simulink model "mdl_example_7_2"  (R2024b)
settings: Solver=FixedStepAuto  StartTime=0.0  StopTime=20*60  FixedStep=1e-2  RelTol=1e-3
values from neighbouring files (symbols this model uses):
  Cd = diag([kd kd kd])    [example_7_2_init.m]
  hw0_B = [0 0 0]'    [example_7_2_init.m]
  inv_qc = inv_q(qc)    [example_7_2_init.m]
  J2 = [6400  -76.4    -25.6 ... (first row only)    [example_7_2_init.m]
  kp = 10    [example_7_2_init.m]
  q0 = (sqrt(2)/2)*[1 0 0 1]'    [example_7_2_init.m]
  w0 = [0.01 0.01 0.01]'    [example_7_2_init.m]
  W4 = (1/sqrt(2))*W4    [example_7_2_init.m]
  W4_inv = pinv(W4)    [example_7_2_init.m]
  WN = [1 0 0 1/sqrt(3) ... (first row only)    [example_7_2_init.m]
  WN_inv = pinv(WN)    [example_7_2_init.m]
libraries: aerolibutil x1
settings Model: SimulationMode=accelerator  Creator=Monster  LastModifiedBy=Monster

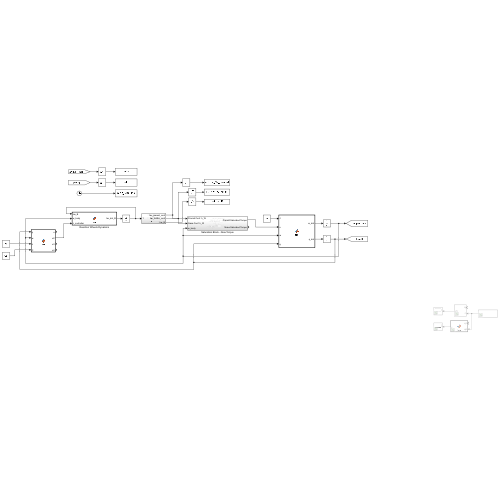
[thumbnail: Simulink's stored preview of the top-level diagram]
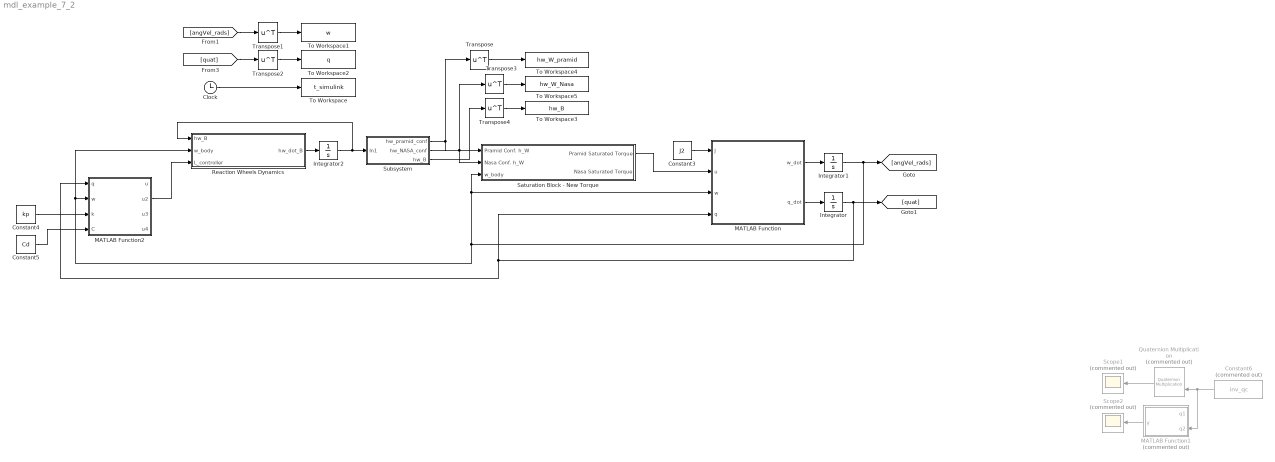
== system mdl_example_7_2 ==
  Clock : Clock
  Constant3 : Constant  Value=J2
  Constant4 : Constant  Value=kp
  Constant5 : Constant  Value=Cd
  Constant6 : Constant  Commented=on  Value=inv_qc
  Integrator : Integrator  InitialCondition=q0
  Integrator1 : Integrator  InitialCondition=w0
  Integrator2 : Integrator  InitialCondition=hw0_B
  MATLAB Function : MATLAB Function  TreatAsAtomicUnit=on
  MATLAB Function1 : MATLAB Function  Commented=on  TreatAsAtomicUnit=on
  MATLAB Function2 : MATLAB Function  TreatAsAtomicUnit=on
  Quaternion Multiplication : aerolibutil/Quaternion Multiplication  Commented=on
  Reaction Wheels Dynamics : MATLAB Function  TreatAsAtomicUnit=on
  Saturation Block - New Torque : Subsystem
  Scope1 : Scope  Commented=on
  Scope2 : Scope  Commented=on
  Subsystem : Subsystem
  To Workspace : ToWorkspace  VariableName=t_simulink  SampleTime=-1
      settings: Save2DSignal=2-D array (concatenate along first dimension)
  To Workspace1 : ToWorkspace  VariableName=w  SampleTime=-1
      settings: Save2DSignal=2-D array (concatenate along first dimension)
  To Workspace2 : ToWorkspace  VariableName=q  SampleTime=-1
      settings: Save2DSignal=2-D array (concatenate along first dimension)
  To Workspace3 : ToWorkspace  VariableName=hw_B  SampleTime=-1
      settings: Save2DSignal=2-D array (concatenate along first dimension)
  To Workspace4 : ToWorkspace  VariableName=hw_W_pramid  SampleTime=-1
      settings: Save2DSignal=2-D array (concatenate along first dimension)
  To Workspace5 : ToWorkspace  VariableName=hw_W_Nasa  SampleTime=-1
      settings: Save2DSignal=2-D array (concatenate along first dimension)
  Transpose{,1..4} (5 alike) : Math  Operator=transpose
  wires:
  MATLAB Function/1(w_dot) -> Integrator1/1
  Integrator1/1 -> [angVel_rads], MATLAB Function2/2(w), Reaction Wheels Dynamics/2(w_body), Saturation Block - New Torque/3(w_body), MATLAB Function/3(w)
  [quat] -> Transpose2/1
  [angVel_rads] -> Transpose1/1
  MATLAB Function/2(q_dot) -> Integrator/1
  Quaternion Multiplication/1 -> Scope1/1
  Constant3/1 -> MATLAB Function/1(J)
  Constant6/1 -> MATLAB Function1/2(q2), Quaternion Multiplication/2
  Constant4/1 -> MATLAB Function2/3(k)
  Constant5/1 -> MATLAB Function2/4(C)
  Integrator/1 -> [quat], MATLAB Function2/1(q), MATLAB Function/4(q)
  MATLAB Function1/1(y) -> Scope2/1
  Clock/1 -> To Workspace/1
  Transpose1/1 -> To Workspace1/1
  Transpose2/1 -> To Workspace2/1
  Reaction Wheels Dynamics/1(hw_dot_B) -> Integrator2/1
  Subsystem/2(hw_NASA_conf) -> Saturation Block - New Torque/2(Nasa Conf. h_W), Transpose3/1
  Subsystem/1(hw_pramid_conf) -> Transpose/1, Saturation Block - New Torque/1(Pramid Conf. h_W)
  Integrator2/1 -> Reaction Wheels Dynamics/1(hw_B), Subsystem/1(In1)
  Transpose3/1 -> To Workspace5/1
  Transpose4/1 -> To Workspace3/1
  Subsystem/3(hw_B) -> Transpose4/1
  Transpose/1 -> To Workspace4/1
  Saturation Block - New Torque/1(Pramid Saturated Torque) -> MATLAB Function/2(u)
  MATLAB Function2/2(u2) -> Reaction Wheels Dynamics/3(L_controller)

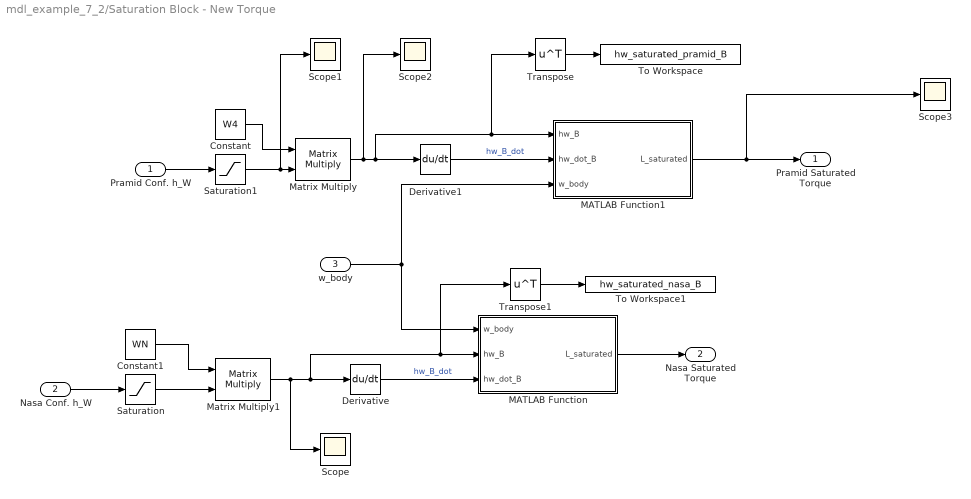
== system mdl_example_7_2/Saturation Block - New Torque ==
  Pramid Conf. h_W : Inport
  Nasa Conf. h_W : Inport  Port=2
  w_body : Inport  Port=3
  Constant : Constant  Value=W4
  Constant1 : Constant  Value=WN
  Derivative : Derivative
  Derivative1 : Derivative
  MATLAB Function : MATLAB Function  TreatAsAtomicUnit=on
  MATLAB Function1 : MATLAB Function  TreatAsAtomicUnit=on
  Matrix Multiply : Product  Multiplication=Matrix(*)
  Matrix Multiply1 : Product  Multiplication=Matrix(*)
  Saturation : Saturate  UpperLimit=250  LowerLimit=-250  LinearizeAsGain=off
  Saturation1 : Saturate  UpperLimit=250  LowerLimit=-250
  Scope{,1..3} (4 alike) : Scope
  To Workspace : ToWorkspace  VariableName=hw_saturated_pramid_B  SampleTime=-1
      settings: Save2DSignal=2-D array (concatenate along first dimension)
  To Workspace1 : ToWorkspace  VariableName=hw_saturated_nasa_B  SampleTime=-1
      settings: Save2DSignal=2-D array (concatenate along first dimension)
  Transpose : Math  Operator=transpose
  Transpose1 : Math  Operator=transpose
  Pramid Saturated Torque : Outport
  Nasa Saturated Torque : Outport  Port=2
  wires:
  Nasa Conf. h_W/1 -> Saturation/1
  Pramid Conf. h_W/1 -> Saturation1/1
  Saturation1/1 -> Scope1/1, Matrix Multiply/2
  Constant/1 -> Matrix Multiply/1
  Saturation/1 -> Matrix Multiply1/2
  Constant1/1 -> Matrix Multiply1/1
  Matrix Multiply1/1 -> Scope/1, Transpose1/1, MATLAB Function/2(hw_B), Derivative/1
  Derivative/1 -> MATLAB Function/3(hw_dot_B)  "hw_B_dot"
  Derivative1/1 -> MATLAB Function1/2(hw_dot_B)  "hw_B_dot"
  Matrix Multiply/1 -> Scope2/1, Transpose/1, MATLAB Function1/1(hw_B), Derivative1/1
  w_body/1 -> MATLAB Function/1(w_body), MATLAB Function1/3(w_body)
  MATLAB Function/1(L_saturated) -> Nasa Saturated Torque/1
  MATLAB Function1/1(L_saturated) -> Scope3/1, Pramid Saturated Torque/1
  Transpose/1 -> To Workspace/1
  Transpose1/1 -> To Workspace1/1

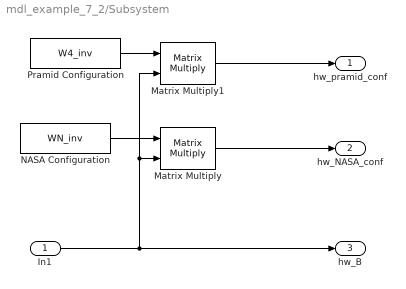
== system mdl_example_7_2/Subsystem ==
  In1 : Inport
  Matrix Multiply : Product  Multiplication=Matrix(*)
  Matrix Multiply1 : Product  Multiplication=Matrix(*)
  NASA Configuration : Constant  Value=WN_inv
  Pramid Configuration : Constant  Value=W4_inv
  hw_pramid_conf : Outport
  hw_NASA_conf : Outport  Port=2
  hw_B : Outport  Port=3
  wires:
  Matrix Multiply/1 -> hw_NASA_conf/1
  Matrix Multiply1/1 -> hw_pramid_conf/1
  Pramid Configuration/1 -> Matrix Multiply1/1
  NASA Configuration/1 -> Matrix Multiply/1
  In1/1 -> hw_B/1, Matrix Multiply1/2, Matrix Multiply/2

== matlab function mdl_example_7_2/MATLAB Function1 ==
  data: q1 input; y output; q2 input
function y = fcn(q1,q2)

y = quat_multip(q1,q2);

== matlab function mdl_example_7_2/MATLAB Function ==
  data: w_dot output; J input; u input; q_dot output; w input; q input
function [w_dot,q_dot] = fcn(J,u,w,q)


w1 = w(1);
w2 = w(2);
w3 = w(3);

W = [ 0,  w3, -w2, w1;
    -w3,   0,  w1, w2;
     w2, -w1,   0, w3;
    -w1, -w2, -w3,  0 ];

% output
w_dot = inv(J)*(u-cross(w,J*w));

q_dot = 0.5*W*q;

end

== matlab function mdl_example_7_2/MATLAB Function2 ==
  data: u output; u2 output; q input; w input; k input; C input; u3 output; u4 output
function [u,u2,u3,u4]= fcn(q,w,k,C)

I3x3 = eye(3,3);
K = k*I3x3;

% Controller I
% Controller II
K2 = k*sign(q(4))*I3x3;
% Controller III
C3 = C*(1+transpose(q(1:3))*q(1:3));
% Controller IIII
C4 = C*(1-transpose(q(1:3))*q(1:3));

u  = -K*q(1:3) - C*w;
u2 = -K2*q(1:3) - C*w;
u3 = -K2*q(1:3) - C3*w;
u4 = -K2*q(1:3) - C4*w;

end

== matlab function mdl_example_7_2/Reaction Wheels Dynamics ==
  data: hw_B input; w_body input; hw_dot_B output; L_controller input
function hw_dot_B = fcn(hw_B, w_body, L_controller)

hw_dot_B = -cross(w_body,hw_B)-L_controller;

end

== matlab function mdl_example_7_2/Saturation Block - New Torque/MATLAB Function ==
  data: w_body input; hw_B input; hw_dot_B input; L_saturated output
function L_saturated = fcn(w_body, hw_B, hw_dot_B)

    L_saturated = -cross(w_body,hw_B) - hw_dot_B;

end

== matlab function mdl_example_7_2/Saturation Block - New Torque/MATLAB Function1 ==
  data: hw_B input; hw_dot_B input; L_saturated output; w_body input
function L_saturated = fcn(hw_B, hw_dot_B, w_body)

    L_saturated = -cross(w_body,hw_B) - hw_dot_B;

end
